simulink model "SmkLim_InjMassLim"  (R2016b)
settings: configuration reference "CodeGenConfigSet" (kept outside this file)
values from neighbouring files (symbols this model uses):
  SmkLim_EGRfacRmpSlopeNeg_C = Calibration.Parameter    [init_SmkLim_InjMassLim.m]    (also in init_SmkLim_InjMassLim_SIL.m = Simulink.Parameter)
  SmkLim_EGRfacRmpSlopePos_C = Calibration.Parameter    [init_SmkLim_InjMassLim.m]    (also in init_SmkLim_InjMassLim_SIL.m = Simulink.Parameter)
  SmkLim_facEnvPCor_CUR = Calibration.Parameter    [init_SmkLim_InjMassLim.m]    (also in init_SmkLim_InjMassLim_SIL.m = Simulink.Parameter)
  SmkLim_facEnvPCor_CURX = Calibration.Parameter    [init_SmkLim_InjMassLim.m]    (also in init_SmkLim_InjMassLim_SIL.m = Simulink.Parameter)
  SmkLim_facLamEGRCor_CUR = Calibration.Parameter    [init_SmkLim_InjMassLim.m]    (also in init_SmkLim_InjMassLim_SIL.m = Simulink.Parameter)
  SmkLim_facLamEGRCor_CURX = Calibration.Parameter    [init_SmkLim_InjMassLim.m]    (also in init_SmkLim_InjMassLim_SIL.m = Simulink.Parameter)
  SmkLim_facStrtCor_CUR = Calibration.Parameter    [init_SmkLim_InjMassLim.m]    (also in init_SmkLim_InjMassLim_SIL.m = Simulink.Parameter)
  SmkLim_facStrtCor_CURX = Calibration.Parameter    [init_SmkLim_InjMassLim.m]    (also in init_SmkLim_InjMassLim_SIL.m = Simulink.Parameter)
  SmkLim_numSmkLim_C = Calibration.Parameter    [init_SmkLim_InjMassLim.m]    (also in init_SmkLim_InjMassLim_SIL.m = Simulink.Parameter)
  SmkLim_rLamEGRCor_MAP = Calibration.Parameter    [init_SmkLim_InjMassLim.m]    (also in init_SmkLim_InjMassLim_SIL.m = Simulink.Parameter)
  SmkLim_rLamEGRCor_MAPX = Calibration.Parameter    [init_SmkLim_InjMassLim.m]    (also in init_SmkLim_InjMassLim_SIL.m = Simulink.Parameter)
  SmkLim_rLamEGRCor_MAPY = Calibration.Parameter    [init_SmkLim_InjMassLim.m]    (also in init_SmkLim_InjMassLim_SIL.m = Simulink.Parameter)
  SmkLim_rLamEnvPCor_MAP = Calibration.Parameter    [init_SmkLim_InjMassLim.m]    (also in init_SmkLim_InjMassLim_SIL.m = Simulink.Parameter)
  SmkLim_rLamEnvPCor_MAPX = Calibration.Parameter    [init_SmkLim_InjMassLim.m]    (also in init_SmkLim_InjMassLim_SIL.m = Simulink.Parameter)
  SmkLim_rLamEnvPCor_MAPY = Calibration.Parameter    [init_SmkLim_InjMassLim.m]    (also in init_SmkLim_InjMassLim_SIL.m = Simulink.Parameter)
  SmkLim_rLamFullLd_MAP = Calibration.Parameter    [init_SmkLim_InjMassLim.m]    (also in init_SmkLim_InjMassLim_SIL.m = Simulink.Parameter)
  SmkLim_rLamFullLd_MAPX = Calibration.Parameter    [init_SmkLim_InjMassLim.m]    (also in init_SmkLim_InjMassLim_SIL.m = Simulink.Parameter)
  SmkLim_rLamFullLd_MAPY = Calibration.Parameter    [init_SmkLim_InjMassLim.m]    (also in init_SmkLim_InjMassLim_SIL.m = Simulink.Parameter)
  SmkLim_rLamMaxEOM_C = Calibration.Parameter    [init_SmkLim_InjMassLim.m]    (also in init_SmkLim_InjMassLim_SIL.m = Simulink.Parameter)
  SmkLim_rLamMinEOM_C = Calibration.Parameter    [init_SmkLim_InjMassLim.m]    (also in init_SmkLim_InjMassLim_SIL.m = Simulink.Parameter)
  SmkLim_rLamSmkEOM0_MAP = Calibration.Parameter    [init_SmkLim_InjMassLim.m]    (also in init_SmkLim_InjMassLim_SIL.m = Simulink.Parameter)
  SmkLim_rLamSmkEOM0_MAPX = Calibration.Parameter    [init_SmkLim_InjMassLim.m]    (also in init_SmkLim_InjMassLim_SIL.m = Simulink.Parameter)
  SmkLim_rLamSmkEOM0_MAPY = Calibration.Parameter    [init_SmkLim_InjMassLim.m]    (also in init_SmkLim_InjMassLim_SIL.m = Simulink.Parameter)
  SmkLim_rLamStrtCor_CUR = Calibration.Parameter    [init_SmkLim_InjMassLim.m]    (also in init_SmkLim_InjMassLim_SIL.m = Simulink.Parameter)
  SmkLim_rLamStrtCor_CURX = Calibration.Parameter    [init_SmkLim_InjMassLim.m]    (also in init_SmkLim_InjMassLim_SIL.m = Simulink.Parameter)
undefined symbols (not defined in the file or in its folder): CEngDsT_tTransf_CURX, SmkLim_InjMassLim_DT, StSys_StrtState_conv
libraries: CXLib x4
settings Model: Creator=xuxingpei  LastModifiedBy=xuxingpei
settings ConfigSetRef: SourceLocation=Base Workspace

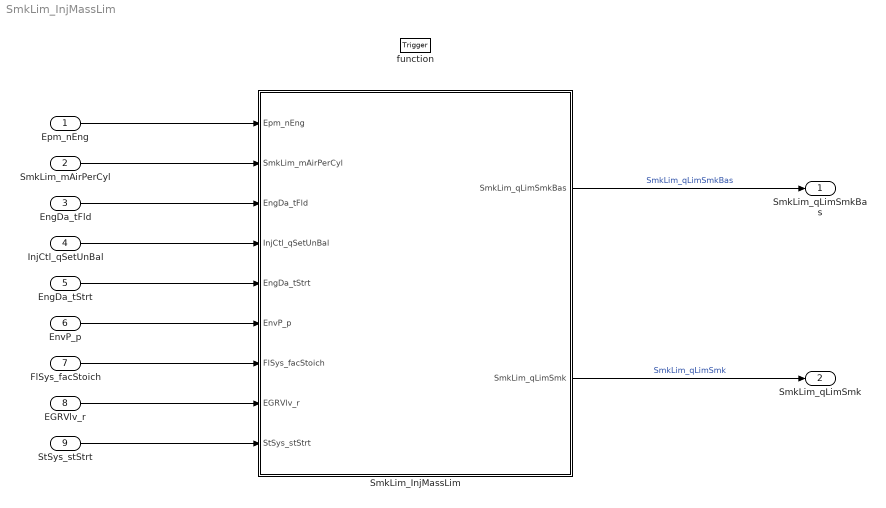
== system SmkLim_InjMassLim ==
  Epm_nEng : Inport  Tag=rpm  Description=Engine speed  OutMin=0  OutMax=6000  OutDataTypeStr=EngSpeed_rpm
  SmkLim_mAirPerCyl : Inport  Tag=mg/hub  Description=Air mass for smoke limitation  Port=2  OutMin=0  OutMax=16383  OutDataTypeStr=AirMass_mg_hub
  EngDa_tFld : Inport  Tag=deg  Description=Engine temperature field  Port=3  OutMin=-3000  OutMax=3000  OutDataTypeStr=Temp_deg  PortDimensions=3
  InjCtl_qSetUnBal : Inport  Tag=mg/hub  Description=Current injection quantity  Port=4  OutMin=-319  OutMax=319  OutDataTypeStr=FuelMass_mg_hub
  EngDa_tStrt : Inport  Tag=deg  Description=Engine starting temperature  Port=5  OutMin=-1000  OutMax=1000  OutDataTypeStr=Temp_deg
  EnvP_p : Inport  Tag=kPa  Description=Barometric pressure  Port=6  OutMin=0  OutMax=3276  OutDataTypeStr=AirPressure_kPa
  FlSys_facStoich : Inport  Description=Stochiometric fuel factor  Port=7  OutMin=-32  OutMax=31  OutDataTypeStr=Factor
  EGRVlv_r : Inport  Tag=%  Description=duty cycle of EGR Valve  Port=8  OutMin=-100  OutMax=100  OutDataTypeStr=Prc_100_rate
  StSys_stStrt : Inport  Description=state of starting system  Port=9  OutDataTypeStr=Enum: StSys_StrtState_conv
  function : TriggerPort  TriggerType=function-call  VariantControl=Variant
  SmkLim_InjMassLim : Subsystem
  SmkLim_qLimSmkBas : Outport  Tag=mg/hub  Description=Smoke limitation quantity in current operation mode  OutMin=-319  OutMax=319  OutDataTypeStr=FuelMass_mg_hub
  SmkLim_qLimSmk : Outport  Tag=mg/hub  Description=Smoke limitation quantity in current operation mode  Port=2  OutMin=-319  OutMax=319  OutDataTypeStr=FuelMass_mg_hub
  wires:
  Epm_nEng/1 -> SmkLim_InjMassLim/1(Epm_nEng)
  SmkLim_mAirPerCyl/1 -> SmkLim_InjMassLim/2(SmkLim_mAirPerCyl)
  EngDa_tFld/1 -> SmkLim_InjMassLim/3(EngDa_tFld)
  InjCtl_qSetUnBal/1 -> SmkLim_InjMassLim/4(InjCtl_qSetUnBal)
  EngDa_tStrt/1 -> SmkLim_InjMassLim/5(EngDa_tStrt)
  EnvP_p/1 -> SmkLim_InjMassLim/6(EnvP_p)
  FlSys_facStoich/1 -> SmkLim_InjMassLim/7(FlSys_facStoich)
  EGRVlv_r/1 -> SmkLim_InjMassLim/8(EGRVlv_r)
  SmkLim_InjMassLim/1(SmkLim_qLimSmkBas) -> SmkLim_qLimSmkBas/1  "SmkLim_qLimSmkBas"
  SmkLim_InjMassLim/2(SmkLim_qLimSmk) -> SmkLim_qLimSmk/1  "SmkLim_qLimSmk"
  StSys_stStrt/1 -> SmkLim_InjMassLim/9(StSys_stStrt)

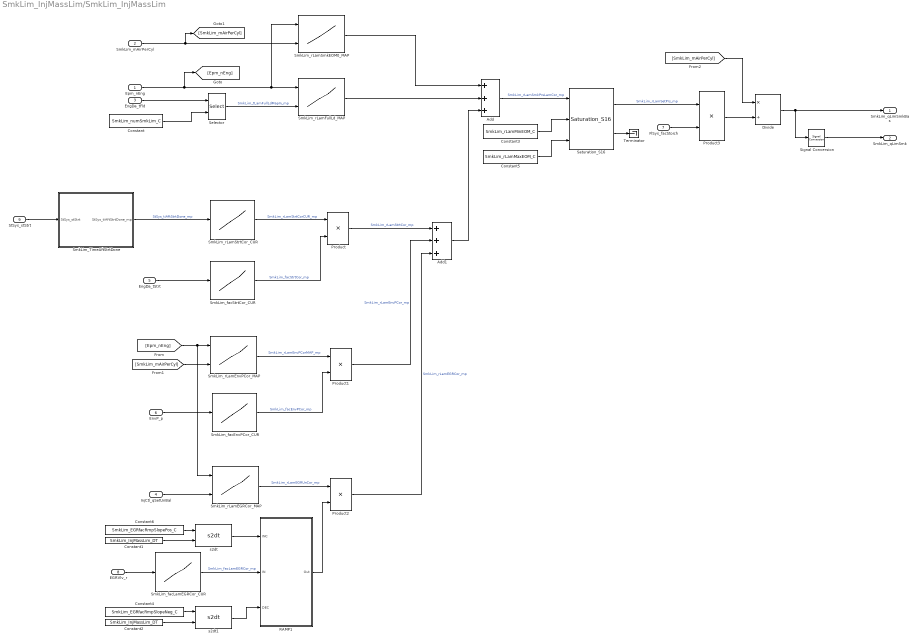
== system SmkLim_InjMassLim/SmkLim_InjMassLim ==
  Epm_nEng : Inport  Tag=rpm  Description=Engine speed  OutMin=0  OutMax=6000  OutDataTypeStr=EngSpeed_rpm
  SmkLim_mAirPerCyl : Inport  Tag=mg/hub  Description=Air mass for smoke limitation  Port=2  OutMin=0  OutMax=16383  OutDataTypeStr=AirMass_mg_hub
  EngDa_tFld : Inport  Tag=deg  Description=Engine temperature field  Port=3  OutMin=-3000  OutMax=3000  OutDataTypeStr=Temp_deg  PortDimensions=3
  InjCtl_qSetUnBal : Inport  Tag=mg/hub  Description=Current injection quantity  Port=4  OutMin=-319  OutMax=319  OutDataTypeStr=FuelMass_mg_hub
  EngDa_tStrt : Inport  Tag=deg  Description=Engine starting temperature  Port=5  OutMin=-1000  OutMax=1000  OutDataTypeStr=Temp_deg
  EnvP_p : Inport  Tag=kPa  Description=Barometric pressure  Port=6  OutMin=0  OutMax=3276  OutDataTypeStr=AirPressure_kPa
  FlSys_facStoich : Inport  Description=Stochiometric fuel factor  Port=7  OutMin=-32  OutMax=31  OutDataTypeStr=Factor
  EGRVlv_r : Inport  Tag=%  Description=duty cycle of EGR Valve  Port=8  OutMin=-100  OutMax=100  OutDataTypeStr=Prc_100_rate
  StSys_stStrt : Inport  Description=state of starting system  Port=9  OutDataTypeStr=Enum: StSys_StrtState_conv
  Add : Sum  Inputs=+++  OutDataTypeStr=Inherit: Inherit via back propagation  SaturateOnIntegerOverflow=on
  Add1 : Sum  Inputs=+++  OutDataTypeStr=Inherit: Inherit via back propagation  SaturateOnIntegerOverflow=on
  Constant : Constant  Value=SmkLim_numSmkLim_C
  Constant1 : Constant  Value=SmkLim_InjMassLim_DT
  Constant2 : Constant  Value=SmkLim_InjMassLim_DT
  Constant3 : Constant  Value=SmkLim_rLamMinEOM_C
  Constant4 : Constant  Value=SmkLim_EGRfacRmpSlopeNeg_C
  Constant5 : Constant  Value=SmkLim_rLamMaxEOM_C
  Constant6 : Constant  Value=SmkLim_EGRfacRmpSlopePos_C
  Divide : Product  Inputs=*/  OutDataTypeStr=Inherit: Inherit via back propagation  SaturateOnIntegerOverflow=on
  Product : Product  OutDataTypeStr=Inherit: Inherit via back propagation  SaturateOnIntegerOverflow=on
  Product1 : Product  OutDataTypeStr=Inherit: Inherit via back propagation  SaturateOnIntegerOverflow=on
  Product2 : Product  OutDataTypeStr=Inherit: Inherit via back propagation  SaturateOnIntegerOverflow=on
  Product3 : Product  SaturateOnIntegerOverflow=on  OutDataTypeStr=Inherit: Same as first input
  RAMP1 : Subsystem
  Saturation_S16 : CXLib/Saturation_S16
  Selector : Selector  IndexMode=Zero-based  InputPortWidth=3  IndexOptions=Index vector (port)  Indices=[1 3]  OutputSizes=1
  Signal Conversion : SignalConversion  OverrideOpt=off
  SmkLim_TimeAftStrtDone : Subsystem
  SmkLim_facEnvPCor_CUR : Lookup_n-D  DialogController=Simulink.DDGSource  NumberOfTableDimensions=1  BreakpointsForDimension1=SmkLim_facEnvPCor_CURX  BreakpointsForDimension2=CEngDsT_tTransf_CURX  IndexSearchMethod=Linear search  BeginIndexSearchUsingPreviousIndexResult=on  Table=SmkLim_facEnvPCor_CUR  ExtrapMethod=Clip  UseLastTableValue=on  InternalRulePriority=Speed  OutDataTypeStr=Inherit: Inherit via back propagation  SaturateOnIntegerOverflow=on
  SmkLim_facLamEGRCor_CUR : Lookup_n-D  DialogController=Simulink.DDGSource  NumberOfTableDimensions=1  BreakpointsForDimension1=SmkLim_facLamEGRCor_CURX  BreakpointsForDimension2=CEngDsT_tTransf_CURX  IndexSearchMethod=Linear search  BeginIndexSearchUsingPreviousIndexResult=on  Table=SmkLim_facLamEGRCor_CUR  ExtrapMethod=Clip  UseLastTableValue=on  InternalRulePriority=Speed  OutDataTypeStr=Inherit: Inherit via back propagation  SaturateOnIntegerOverflow=on
  SmkLim_facStrtCor_CUR : Lookup_n-D  DialogController=Simulink.DDGSource  NumberOfTableDimensions=1  BreakpointsForDimension1=SmkLim_facStrtCor_CURX  BreakpointsForDimension2=CEngDsT_tTransf_CURX  IndexSearchMethod=Linear search  BeginIndexSearchUsingPreviousIndexResult=on  Table=SmkLim_facStrtCor_CUR  ExtrapMethod=Clip  UseLastTableValue=on  InternalRulePriority=Speed  OutDataTypeStr=Inherit: Inherit via back propagation  SaturateOnIntegerOverflow=on
  SmkLim_rLamEGRCor_MAP : Lookup_n-D  BreakpointsForDimension1=SmkLim_rLamEGRCor_MAPY  BreakpointsForDimension2=SmkLim_rLamEGRCor_MAPX  IndexSearchMethod=Linear search  BeginIndexSearchUsingPreviousIndexResult=on  Table=SmkLim_rLamEGRCor_MAP  ExtrapMethod=Clip  UseLastTableValue=on  InternalRulePriority=Speed  OutDataTypeStr=Inherit: Inherit via back propagation  RndMeth=Simplest  SaturateOnIntegerOverflow=on
  SmkLim_rLamEnvPCor_MAP : Lookup_n-D  BreakpointsForDimension1=SmkLim_rLamEnvPCor_MAPY  BreakpointsForDimension2=SmkLim_rLamEnvPCor_MAPX  IndexSearchMethod=Linear search  BeginIndexSearchUsingPreviousIndexResult=on  Table=SmkLim_rLamEnvPCor_MAP  ExtrapMethod=Clip  UseLastTableValue=on  InternalRulePriority=Speed  OutDataTypeStr=Inherit: Inherit via back propagation  RndMeth=Simplest  SaturateOnIntegerOverflow=on
  SmkLim_rLamFullLd_MAP : Lookup_n-D  BreakpointsForDimension1=SmkLim_rLamFullLd_MAPY  BreakpointsForDimension2=SmkLim_rLamFullLd_MAPX  IndexSearchMethod=Linear search  BeginIndexSearchUsingPreviousIndexResult=on  Table=SmkLim_rLamFullLd_MAP  ExtrapMethod=Clip  UseLastTableValue=on  InternalRulePriority=Speed  OutDataTypeStr=Inherit: Inherit via back propagation  RndMeth=Simplest  SaturateOnIntegerOverflow=on
  SmkLim_rLamSmkEOM0_MAP : Lookup_n-D  BreakpointsForDimension1=SmkLim_rLamSmkEOM0_MAPY  BreakpointsForDimension2=SmkLim_rLamSmkEOM0_MAPX  IndexSearchMethod=Linear search  BeginIndexSearchUsingPreviousIndexResult=on  Table=SmkLim_rLamSmkEOM0_MAP  ExtrapMethod=Clip  UseLastTableValue=on  InternalRulePriority=Speed  OutDataTypeStr=Inherit: Inherit via back propagation  RndMeth=Simplest  SaturateOnIntegerOverflow=on
  SmkLim_rLamStrtCor_CUR : Lookup_n-D  DialogController=Simulink.DDGSource  NumberOfTableDimensions=1  BreakpointsForDimension1=SmkLim_rLamStrtCor_CURX  BreakpointsForDimension2=CEngDsT_tTransf_CURX  IndexSearchMethod=Linear search  BeginIndexSearchUsingPreviousIndexResult=on  Table=SmkLim_rLamStrtCor_CUR  ExtrapMethod=Clip  UseLastTableValue=on  InternalRulePriority=Speed  OutDataTypeStr=Inherit: Inherit via back propagation  SaturateOnIntegerOverflow=on
  Terminator : Terminator
  s2dt : CXLib/s2dt
  s2dt1 : CXLib/s2dt
  SmkLim_qLimSmkBas : Outport  Tag=mg/hub  Description=Smoke limitation quantity in current operation mode  OutMin=-319  OutMax=319  OutDataTypeStr=FuelMass_mg_hub
  SmkLim_qLimSmk : Outport  Tag=mg/hub  Description=Smoke limitation quantity in current operation mode  Port=2  OutMin=-319  OutMax=319  OutDataTypeStr=FuelMass_mg_hub
  wires:
  SmkLim_facLamEGRCor_CUR/1 -> RAMP1/2(IN)  "SmkLim_facLamEGRCor_mp"
  EngDa_tFld/1 -> Selector/1
  EnvP_p/1 -> SmkLim_facEnvPCor_CUR/1
  SmkLim_facEnvPCor_CUR/1 -> Product1/2  "SmkLim_facEnvPCor_mp"
  Product2/1 -> Add1/3  "SmkLim_rLamEGRCor_mp"
  [Epm_nEng] -> SmkLim_rLamEGRCor_MAP/1, SmkLim_rLamEnvPCor_MAP/1
  EGRVlv_r/1 -> SmkLim_facLamEGRCor_CUR/1
  SmkLim_rLamEGRCor_MAP/1 -> Product2/1  "SmkLim_rLamEGRUnCor_mp"
  Product3/1 -> Divide/2
  Constant/1 -> Selector/2
  [SmkLim_mAirPerCyl] -> Divide/1
  [SmkLim_mAirPerCyl] -> SmkLim_rLamEnvPCor_MAP/2
  Product/1 -> Add1/1  "SmkLim_rLamStrtCor_mp"
  Add1/1 -> Add/3
  Signal Conversion/1 -> SmkLim_qLimSmk/1
  s2dt/1 -> RAMP1/1(INC)
  SmkLim_facStrtCor_CUR/1 -> Product/2  "SmkLim_facStrtCor_mp"
  Constant1/1 -> s2dt/2
  Selector/1 -> SmkLim_rLamFullLd_MAP/2  "SmkLim_tLamFullLdMapIn_mp"
  Epm_nEng/1 -> SmkLim_rLamSmkEOM0_MAP/1, SmkLim_rLamFullLd_MAP/1, [Epm_nEng]
  RAMP1/1(Out) -> Product2/2
  Divide/1 -> SmkLim_qLimSmkBas/1, Signal Conversion/1
  EngDa_tStrt/1 -> SmkLim_facStrtCor_CUR/1
  SmkLim_rLamEnvPCor_MAP/1 -> Product1/1  "SmkLim_rLamEnvPCorMAP_mp"
  SmkLim_mAirPerCyl/1 -> SmkLim_rLamSmkEOM0_MAP/2, [SmkLim_mAirPerCyl]
  SmkLim_rLamStrtCor_CUR/1 -> Product/1  "SmkLim_rLamStrtCorCUR_mp"
  Product1/1 -> Add1/2  "SmkLim_rLamEnvPCor_mp"
  InjCtl_qSetUnBal/1 -> SmkLim_rLamEGRCor_MAP/2
  Constant6/1 -> s2dt/1
  Constant5/1 -> Saturation_S16/3
  s2dt1/1 -> RAMP1/3(DEC)
  Saturation_S16/2 -> Terminator/1
  Constant2/1 -> s2dt1/2
  Constant4/1 -> s2dt1/1
  Constant3/1 -> Saturation_S16/2
  Add/1 -> Saturation_S16/1  "SmkLim_rLamSmkPrsLamCor_mp"
  StSys_stStrt/1 -> SmkLim_TimeAftStrtDone/1(StSys_stStrt)
  SmkLim_TimeAftStrtDone/1(StSys_tiAftStrtDone_mp) -> SmkLim_rLamStrtCor_CUR/1  "StSys_tiAftStrtDone_mp"
  SmkLim_rLamFullLd_MAP/1 -> Add/2
  SmkLim_rLamSmkEOM0_MAP/1 -> Add/1
  Saturation_S16/1 -> Product3/1  "SmkLim_rLamSetPrs_mp"
  FlSys_facStoich/1 -> Product3/2

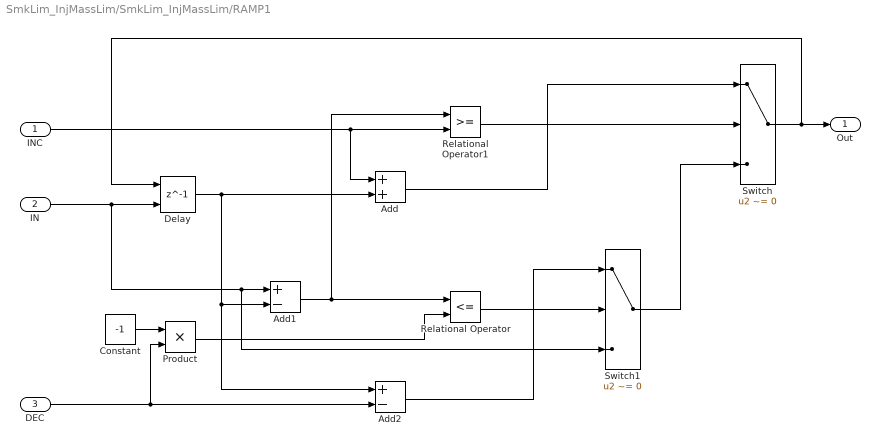
== system SmkLim_InjMassLim/SmkLim_InjMassLim/RAMP1 ==
  INC : Inport
  IN : Inport  Port=2
  DEC : Inport  Port=3
  Add : Sum  SaturateOnIntegerOverflow=on  InputSameDT=on
  Add1 : Sum  Inputs=+-  InputSameDT=on
  Add2 : Sum  Inputs=+-  SaturateOnIntegerOverflow=on  InputSameDT=on
  Constant : Constant  Value=-1  OutDataTypeStr=Inherit: Inherit via back propagation
  Delay : Delay  DelayLength=1  InitialConditionSource=Input port
      settings: InputPortMap=u0,p4
  Product : Product  OutDataTypeStr=Inherit: Inherit via back propagation  InputSameDT=on
  Relational Operator : RelationalOperator  Operator=<=  OutDataTypeStr=boolean  RndMeth=Simplest  InputSameDT=on
  Relational Operator1 : RelationalOperator  OutDataTypeStr=boolean  RndMeth=Simplest
  Switch : Switch  Criteria=u2 ~= 0
  Switch1 : Switch  Criteria=u2 ~= 0
  Out : Outport
  wires:
  IN/1 -> Switch1/3, Add1/1, Delay/2
  Delay/1 -> Add2/1, Add1/2, Add/2
  Add1/1 -> Relational Operator1/1, Relational Operator/1
  INC/1 -> Add/1, Relational Operator1/2
  Relational Operator1/1 -> Switch/2
  Add/1 -> Switch/1
  Switch/1 -> Delay/1, Out/1
  Relational Operator/1 -> Switch1/2
  Switch1/1 -> Switch/3
  Constant/1 -> Product/1
  DEC/1 -> Product/2, Add2/2
  Product/1 -> Relational Operator/2
  Add2/1 -> Switch1/1

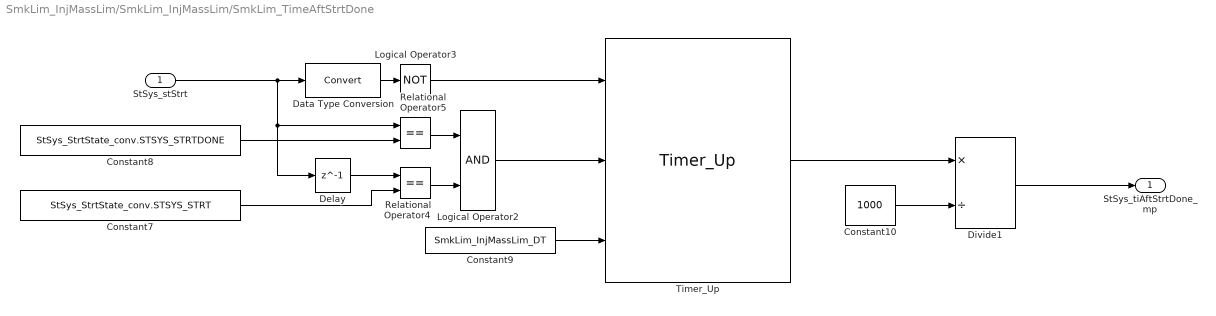
== system SmkLim_InjMassLim/SmkLim_InjMassLim/SmkLim_TimeAftStrtDone ==
  StSys_stStrt : Inport  Description=state of starting system  OutDataTypeStr=Enum: StSys_StrtState_conv
  Constant10 : Constant  Value=1000  OutDataTypeStr=Inherit: Inherit via back propagation
  Constant7 : Constant  Value=StSys_StrtState_conv.STSYS_STRT
  Constant8 : Constant  Value=StSys_StrtState_conv.STSYS_STRTDONE
  Constant9 : Constant  Value=SmkLim_InjMassLim_DT
  Data Type Conversion : DataTypeConversion
  Delay : Delay  DelayLength=1  InitialCondition=StSys_StrtState_conv.STSYS_STRTDONE
  Divide1 : Product  Inputs=*/  OutDataTypeStr=Inherit: Inherit via back propagation
  Logical Operator2 : Logic  AllPortsSameDT=off  OutDataTypeStr=boolean
  Logical Operator3 : Logic  Operator=NOT  AllPortsSameDT=off  OutDataTypeStr=boolean
  Relational Operator4 : RelationalOperator  Operator===  OutDataTypeStr=boolean  RndMeth=Simplest
  Relational Operator5 : RelationalOperator  Operator===  OutDataTypeStr=boolean  RndMeth=Simplest
  Timer_Up : CXLib/Timer_Up
  StSys_tiAftStrtDone_mp : Outport
  wires:
  StSys_stStrt/1 -> Delay/1, Relational Operator5/1, Data Type Conversion/1
  Delay/1 -> Relational Operator4/1
  Constant7/1 -> Relational Operator4/2
  Constant8/1 -> Relational Operator5/2
  Relational Operator5/1 -> Logical Operator2/1
  Relational Operator4/1 -> Logical Operator2/2
  Logical Operator2/1 -> Timer_Up/2
  Constant9/1 -> Timer_Up/3
  Data Type Conversion/1 -> Logical Operator3/1
  Timer_Up/1 -> Divide1/1
  Logical Operator3/1 -> Timer_Up/1
  Divide1/1 -> StSys_tiAftStrtDone_mp/1
  Constant10/1 -> Divide1/2
